simulink model "mc_AdaptiveThreshold"  (R2020a)
settings: Solver=VariableStepAuto  StartTime=0.0  StopTime=10  RelTol=1e-3
undefined symbols (not defined in the file): feature_gain, fs
libraries: dspswit3 x1, dspstat3 x1, simulink x1
settings Model: Creator=sbuccelli  LastModifiedBy=diflo

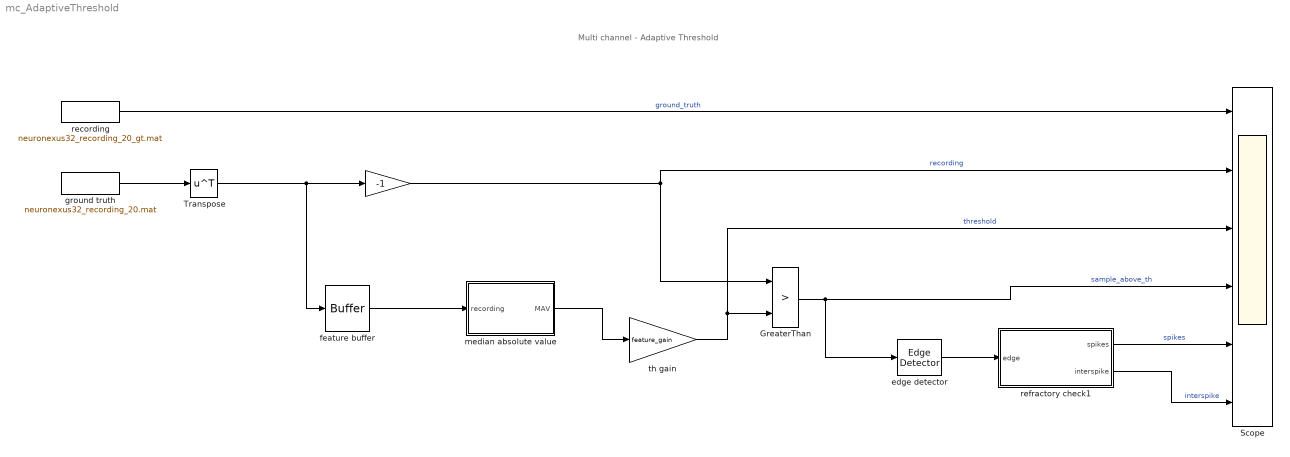
== system mc_AdaptiveThreshold ==
  note: Multi channel - Adaptive Threshold
  " " : Gain  Gain=-1
  GreaterThan : RelationalOperator  Operator=>  OutDataTypeStr=boolean  RndMeth=Simplest
  Scope : Scope  NumInputPorts=6
  Transpose : Math  Operator=transpose  SaturateOnIntegerOverflow=on
  edge detector : dspswit3/Edge Detector  InputProcessing=Columns as channels (frame based)
      settings: SourceProductBaseCode=DS
  feature buffer : Buffer  N=32000  OutputFrames=off
  ground truth : FromFile  FileName=neuronexus32_recording_20.mat  SampleTime=1/fs
  median absolute value : Subsystem
  recording : FromFile  FileName=neuronexus32_recording_20_gt.mat  SampleTime=1/fs
  refractory check1 : Subsystem
  th gain : Gain  Gain=feature_gain
  wires:
  recording/1 -> Scope/1  "ground_truth"
  edge detector/1 -> refractory check1/1("edge  ")
  refractory check1/2(interspike) -> Scope/6  "interspike"
  GreaterThan/1 -> Scope/4, edge detector/1  "sample_above_th"
  th gain/1 -> GreaterThan/2, Scope/3  "threshold"
  refractory check1/1(spikes) -> Scope/5  "spikes"
  ground truth/1 -> Transpose/1
  " "/1 -> GreaterThan/1, Scope/2  "recording"
  feature buffer/1 -> median absolute value/1(recording)
  median absolute value/1(MAV) -> th gain/1
  Transpose/1 -> feature buffer/1, " "/1

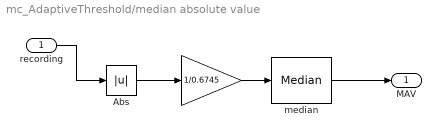
== system mc_AdaptiveThreshold/median absolute value ==
  recording : Inport
  "  " : Gain  Gain=1/0.6745
  Abs : Abs
  median : dspstat3/Median  sortAlg=Quick sort  directionMode=Each column  dimension=1  roundingMode=Floor  overflowMode=off  accumDataTypeStr=Inherit: Same as product output  accumLastDataTypeStr=Inherit: Same as product output  outputDataTypeStr=Inherit: Same as accumulator  outputMin=[]  outputMax=[]  outputLastDataTypeStr=Inherit: Same as accumulator
      settings: SourceProductBaseCode=DS  allowOverrides=off
  MAV : Outport
  wires:
  Abs/1 -> "  "/1
  "  "/1 -> median/1
  recording/1 -> Abs/1
  median/1 -> MAV/1

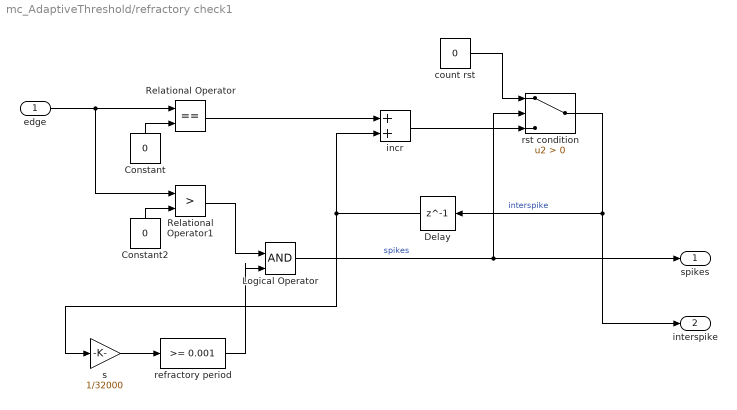
== system mc_AdaptiveThreshold/refractory check1 ==
  "edge  " : Inport
  Constant : Constant  Value=0
  Constant2 : Constant  Value=0
  Delay : Delay  DelayLength=1  InitialCondition=1
  Logical Operator : Logic  IconShape=distinctive  AllPortsSameDT=off  OutDataTypeStr=boolean
  Relational Operator : RelationalOperator  Operator===  OutDataTypeStr=boolean  RndMeth=Simplest
  Relational Operator1 : RelationalOperator  Operator=>  OutDataTypeStr=boolean  RndMeth=Simplest
  count rst : Constant  Value=0
  incr : Sum  AccumDataTypeStr=double
  refractory period : simulink/Logic and Bit Operations/Compare To Constant  relop=>=  const=0.001  OutDataTypeStr=boolean
  rst condition : Switch  Criteria=u2 > Threshold  OutDataTypeStr=double
  s : Gain  Gain=1/32000
  spikes : Outport
  interspike : Outport  Port=2
  wires:
  count rst/1 -> rst condition/1
  Constant/1 -> Relational Operator/2
  Constant2/1 -> Relational Operator1/2
  Relational Operator1/1 -> Logical Operator/1
  refractory period/1 -> Logical Operator/2
  Logical Operator/1 -> spikes/1, rst condition/2  "spikes"
  incr/1 -> rst condition/3
  rst condition/1 -> interspike/1, Delay/1  "interspike"
  Delay/1 -> s/1, incr/2
  Relational Operator/1 -> incr/1
  "edge  "/1 -> Relational Operator1/1, Relational Operator/1
  s/1 -> refractory period/1
